simulink model "torque_control_SIL"  (R2023b)
settings: Solver=FixedStepAuto  StartTime=0.0  StopTime=10  RelTol=1e-3  EnableMultiTasking=on
settings Model: SILPILSystemUnderTest=refmodels  ExtModeTrigDuration=10  Creator=miche  LastModifiedBy=miche
settings OptimizationCC: EnhancedBackFolding=on  PassReuseOutputArgsAs=Individual arguments  ZeroExternalMemoryAtStartup=off  ZeroInternalMemoryAtStartup=off  MaxStackSize=64  OptimizeBlockOrder=speed  DifferentSizesBufferReuse=on  OptimizationCustomize=off  EfficientTunableParamExpr=on
settings DebuggingCC: ParameterTunabilityLossMsg=error
settings HardwareCC: ProdBitPerPointer=32  ProdBitPerSizeT=32  ProdBitPerPtrDiffT=32  ProdLargestAtomicInteger=Long  ProdLargestAtomicFloat=Double  ProdWordSize=32  ProdLongLongMode=on  ProdHWDeviceType=ARM Compatible->ARM Cortex
settings SFSimCC: MATLABDynamicMemAlloc=off
settings RTWCC: Description=Embedded Coder  SystemTargetFile=ert.tlc  HardwareBoard=STM32 Nucleo F401RE  TemplateMakefile=ert_default_tmf  Toolchain=LCC-win64 v2.4.1 | gmake (64-bit Windows)  PortableWordSizes=on  CodeExecutionProfiling=on
settings CodeAppCC: ForceParamTrailComments=on  IgnoreCustomStorageClasses=off  OperatorAnnotations=on  SimulinkDataObjDesc=on  SFDataObjDesc=on  InsertBlockDesc=on
settings ERTTargetCC: ExtModeTransport=3  ExtModeStaticAlloc=on  ExtModeStaticAllocSize=2000  ExtModeMexFile=ext_xcp  ExtModeIntrfLevel=Level2 - Open

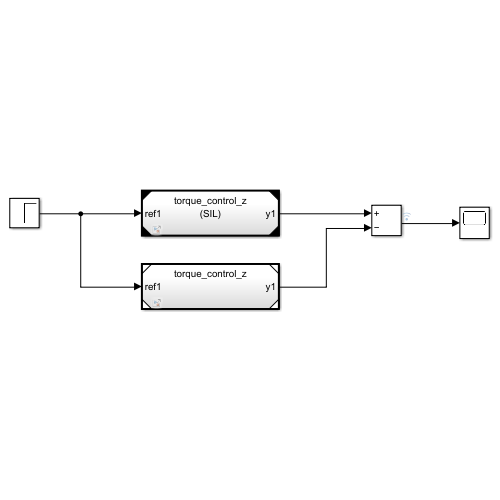
[thumbnail: Simulink's stored preview of the top-level diagram]
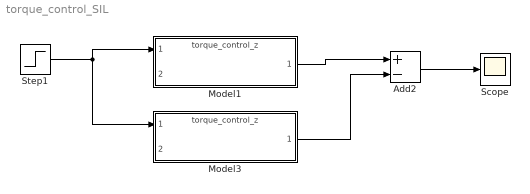
== system torque_control_SIL ==
  Add2 : Sum  Inputs=+-
  Model1 : ModelReference  ModelNameDialog=torque_control_z.slx  SimulationMode=Software-in-the-loop (SIL)  ModelReferenceVersion=1.182
  Model3 : ModelReference  ModelNameDialog=torque_control_z.slx  SimulationMode=Normal  ModelReferenceVersion=1.182
  Scope : Scope
  Step1 : Step  Time=3  After=0.15
  wires:
  Model1/1 -> Add2/1
  Add2/1 -> Scope/1
  Step1/1 -> Model3/1, Model1/1
  Model3/1 -> Add2/2
